simulink model "SSMM_sim_Torque_3DOF"  (R2021a)
settings: Solver=FixedStepAuto  StartTime=0.0  StopTime=15  FixedStep=0.001  MaxStep=1e-1  MinStep=1e-6  RelTol=.05  AbsTol=.05  EnableMultiTasking=on
InitFcn:
  | SSMM_sim_Torque_3DOF_Init
values from neighbouring files (symbols this model uses):
  angVeloSat = 4    [prerun.m]
  CP_Num = CP_Base_Num + CP_Wheels_Num    [JACKAL_dynamic_model.m]
  D = 1000    [JACKAL_dynamic_model.m]
  delay = 0.075    [JACKAL_dynamic_model.m]
  K = 1000000    [JACKAL_dynamic_model.m]
  kd = -0.002    [JACKAL_dynamic_model.m]
  ki = 500    [JACKAL_dynamic_model.m]
  kp = 4    [JACKAL_dynamic_model.m]
  model = floatbase(model)    [JACKAL_dynamic_model.m]
  Mu = .85    (= 0.85)    [JACKAL_dynamic_model.m]
  path = waypoints    [AutoRun.m]
  q_init = [0 0 0 0]'    [JACKAL_dynamic_model.m]
  qd_init = [0 0 0 0]'    [JACKAL_dynamic_model.m]
  realistic_linear_velocity_factor = 0.9782    [JACKAL_dynamic_model.m]
  speed = 2    [prerun.m]
  torque_saturation = 7    [JACKAL_dynamic_model.m]
  wheel_radius = .098    (= 0.098)    [JACKAL_dynamic_model.m]
  wheel_veocity_saturation = 2.2    [JACKAL_dynamic_model.m]
  x_init = [1 0 0 0  0 0 zoff   0 0 0  0 0 0]'    [JACKAL_dynamic_model.m]
undefined symbols (not defined in the file or in its folder): DiscIntNeverNeededParam, Fpt, gcontact, gcPosVel
libraries: simulink x8, fuzblock x3, robotalgslib x1
settings Model: Creator=Sergio  LastModifiedBy=auvsl
settings SolverCC: MaxConsecutiveMinStep=5  AlgebraicLoopSolver=TrustRegion
settings DataIOCC: SaveFormat=Array  SignalLoggingSaveFormat=ModelDataLogs  ReturnWorkspaceOutputs=off
settings OptimizationCC: ExpressionDepthLimit=2147483647  LifeSpan=inf
settings DebuggingCC: UnderspecifiedInitializationDetection=Classic  MergeDetectMultiDrivingBlocksExec=none  SolverPrmCheckMsg=warning  MultiTaskDSMMsg=warning  MultiTaskCondExecSysMsg=none  StateNameClashWarn=warning  SFUnexpectedBacktrackingDiag=warning  SFNoUnconditionalDefaultTransitionDiag=warning  SFExecutionAtInitializationDiag=none  SFMachineParentedDataDiag=warning  ArithmeticOperatorsInVariantConditions=warning
settings HardwareCC: ProdBitPerPointer=32  ProdBitPerSizeT=32  ProdBitPerPtrDiffT=32  ProdLargestAtomicFloat=None  ProdIntDivRoundTo=Undefined  ProdEndianess=Unspecified  ProdWordSize=32  ProdHWDeviceType=32-bit Generic
settings ModelReferenceCC: PropagateSignalLabelsOutOfModel=off
settings SFSimCC: SimUseLocalCustomCode=off  CustomCodeUndefinedFunction=UseInterfaceOnly
settings RTWCC: RTWUseLocalCustomCode=off
settings CodeAppCC: StateflowObjectComments=on
settings GRTTargetCC: TargetLangStandard=C89/C90 (ANSI)
settings ConfigComp: CovMetricSettings=dw  CovSaveCumulativeToWorkspaceVar=on  CovSaveSingleToWorkspaceVar=on  CovExternalEMLEnable=off

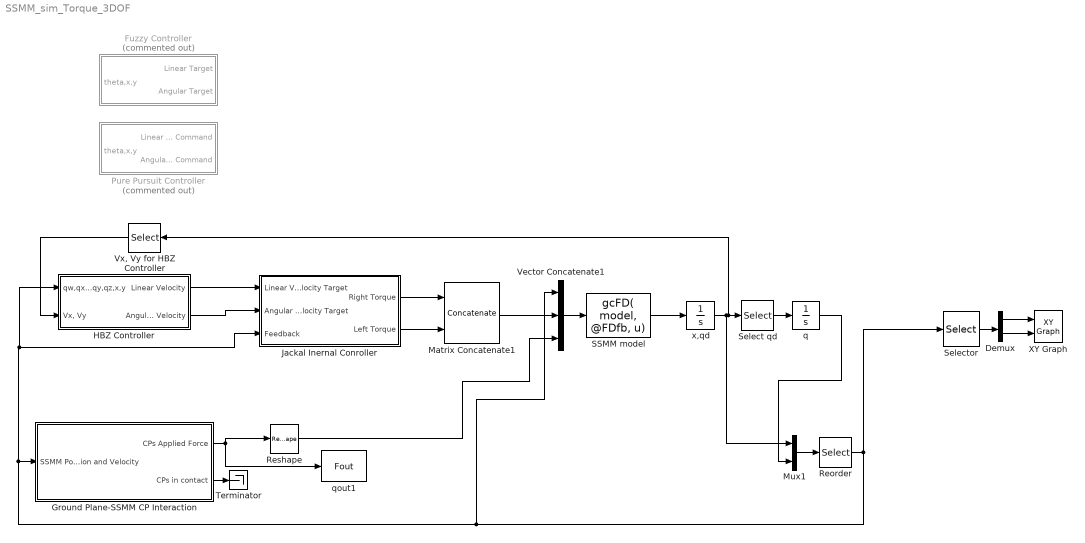
== system SSMM_sim_Torque_3DOF ==
  Demux : Demux  Outputs=2
  Fuzzy Controller : Subsystem  Commented=on
  Ground Plane-SSMM CP Interaction : Subsystem
  HBZ Controller : Subsystem
  Jackal Inernal Conroller : Subsystem
  Matrix Concatenate1 : Concatenate  Mode=Multidimensional array
  Mux1 : Mux  Inputs=2
  Pure Pursuit Controller : Subsystem  Commented=on
  Reorder : Selector  InputPortWidth=21  IndexOptions=Index vector (dialog)  Indices=[1 2 3 4 5 6 7 8 9 10 11 12 13 18 19 20 21 14 15 16 17]  OutputSizes=1
  Reshape : Reshape  OutputDimensionality=Column vector (2-D)
  SSMM model : MATLABFcn  MATLABFcn=gcFD( model, @FDfb, u)  OutputDimensions=[17 1]  OutputSignalType=real  Output1D=off
  Select qd : Selector  InputPortWidth=17  IndexOptions=Index vector (dialog)  Indices=[14 15 16 17]  OutputSizes=1
  Selector : Selector  InputPortWidth=21  IndexOptions=Index vector (dialog)  Indices=[5 6]  OutputSizes=1
  Terminator : Terminator
  Vector Concatenate1 : Concatenate  NumInputs=3
  "Vx, Vy for HBZ Controller" : Selector  InputPortWidth=17  IndexOptions=Index vector (dialog)  Indices=[5, 6]  OutputSizes=1
  XY Graph : simulink/Sinks/XY Graph  xmin=0  xmax=20  ymin=-10  ymax=10  st=-1
  q : Integrator  InitialCondition=q_init
  qout1 : ToWorkspace  VariableName=Fout  SampleTime=-1
  x,qd : Integrator  InitialCondition=[x_init;qd_init]
  wires:
  Vector Concatenate1/1 -> SSMM model/1
  SSMM model/1 -> x,qd/1
  Reshape/1 -> Vector Concatenate1/3
  x,qd/1 -> "Vx, Vy for HBZ Controller"/1, Select qd/1, Mux1/1
  Select qd/1 -> q/1
  Mux1/1 -> Reorder/1
  q/1 -> Mux1/2
  Ground Plane-SSMM CP Interaction/1(CPs Applied Force) -> Reshape/1, qout1/1
  Matrix Concatenate1/1 -> Vector Concatenate1/2
  Jackal Inernal Conroller/1(Right Torque) -> Matrix Concatenate1/1
  Jackal Inernal Conroller/2(Left Torque) -> Matrix Concatenate1/2
  Demux/2 -> XY Graph/2
  Selector/1 -> Demux/1
  Demux/1 -> XY Graph/1
  Ground Plane-SSMM CP Interaction/2(CPs in contact) -> Terminator/1
  Reorder/1 -> Vector Concatenate1/1, HBZ Controller/1(qw,qx,qy,qz,x,y), Jackal Inernal Conroller/3(Feedback), Ground Plane-SSMM CP Interaction/1(SSMM Position and Velocity), Selector/1
  HBZ Controller/1(Linear Velocity) -> Jackal Inernal Conroller/1(Linear Velocity Target)
  HBZ Controller/2(Angular Velocity) -> Jackal Inernal Conroller/2(Angular Velocity Target)
  "Vx, Vy for HBZ Controller"/1 -> HBZ Controller/2("Vx, Vy")

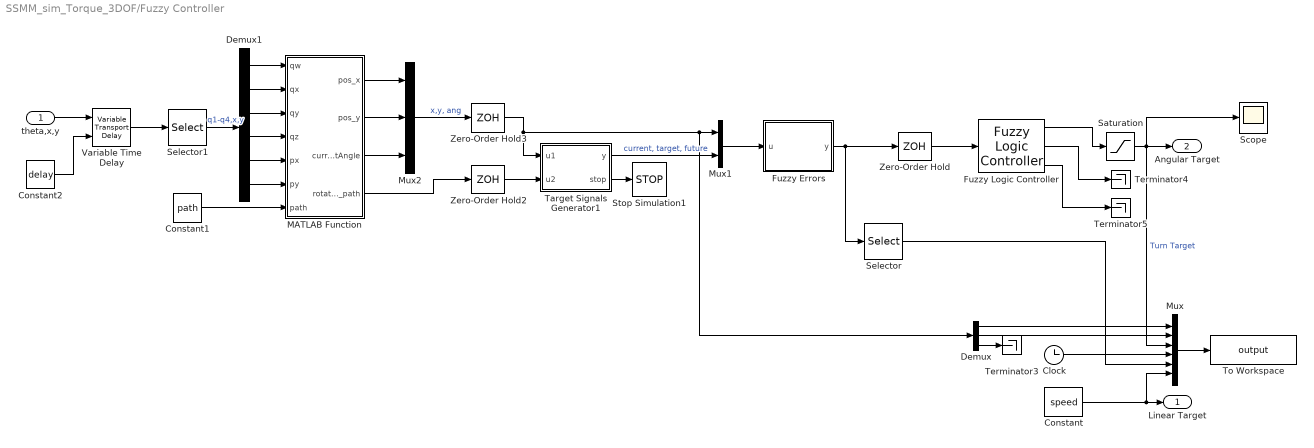
== system SSMM_sim_Torque_3DOF/Fuzzy Controller ==
  theta,x,y : Inport
  Clock : Clock
  Constant : Constant  Value=speed
  Constant1 : Constant  Value=path
  Constant2 : Constant  Value=delay
  Demux : Demux  Outputs=3
  Demux1 : Demux  Outputs=6
  Fuzzy Errors : MATLAB Function  TreatAsAtomicUnit=on
  Fuzzy Logic Controller : fuzblock/Fuzzy Logic  Controller  FIS='fuzV1.fis'  OutputSampleNumber=3000  DataType=double  FuzzifiedInputs=off  RuleFiringStrengths=on  RuleOutputs=off  AggregatedOutputs=on  SimulateUsing=Code generation  OutOfRangeInputValueMessage=warning  NoRuleFiredMessage=warning  EmptyOutputFuzzySetMessage=warning
  MATLAB Function : MATLAB Function  TreatAsAtomicUnit=on
  Mux : Mux  Inputs=6
  Mux1 : Mux  Inputs=2
  Mux2 : Mux  Inputs=3
  Saturation : Saturate  UpperLimit=angVeloSat  LowerLimit=-angVeloSat
  Scope : Scope
  Selector : Selector  InputPortWidth=5  IndexOptions=Index vector (dialog)  Indices=[1]  OutputSizes=1
  Selector1 : Selector  InputPortWidth=21  IndexOptions=Index vector (dialog)  Indices=[1 2 3 4 5 6]  OutputSizes=1
  Stop Simulation1 : Stop
  Target Signals Generator1 : MATLAB Function  TreatAsAtomicUnit=on
  Terminator3 : Terminator
  Terminator4 : Terminator
  Terminator5 : Terminator
  To Workspace : ToWorkspace  VariableName=output  SampleTime=-1
  Variable Time Delay : VariableTransportDelay  MaximumDelay=10  MaximumPoints=6244
  Zero-Order Hold : ZeroOrderHold  SampleTime=.001
  Zero-Order Hold2 : ZeroOrderHold  SampleTime=.001
  Zero-Order Hold3 : ZeroOrderHold  SampleTime=.001
  Linear Target : Outport  VectorParamsAs1DForOutWhenUnconnected=off
  " Angular Target" : Outport  Port=2  VectorParamsAs1DForOutWhenUnconnected=off
  wires:
  Mux1/1 -> Fuzzy Errors/1(u)
  Target Signals Generator1/1(y) -> Mux1/2  "current, target, future"
  Zero-Order Hold2/1 -> Target Signals Generator1/2(u2)
  Target Signals Generator1/2(stop) -> Stop Simulation1/1
  Fuzzy Errors/1(y) -> Selector/1, Zero-Order Hold/1
  Zero-Order Hold/1 -> Fuzzy Logic Controller/1
  Fuzzy Logic Controller/1 -> Saturation/1
  Saturation/1 -> Scope/1, Mux/3, " Angular Target"/1  "Turn Target"
  theta,x,y/1 -> Variable Time Delay/1
  Variable Time Delay/1 -> Selector1/1
  Constant/1 -> Mux/6, Linear Target/1
  Selector/1 -> Mux/5
  Mux/1 -> To Workspace/1
  Zero-Order Hold3/1 -> Target Signals Generator1/1(u1), Mux1/1, Demux/1
  Constant2/1 -> Variable Time Delay/2
  Clock/1 -> Mux/4
  Fuzzy Logic Controller/2 -> Terminator4/1
  Fuzzy Logic Controller/3 -> Terminator5/1
  MATLAB Function/3(currentAngle) -> Mux2/3
  MATLAB Function/1(pos_x) -> Mux2/1
  MATLAB Function/2(pos_y) -> Mux2/2
  MATLAB Function/4(rotated_path) -> Zero-Order Hold2/1
  Mux2/1 -> Zero-Order Hold3/1  "x,y, ang"
  Constant1/1 -> MATLAB Function/7(path)
  Demux1/1 -> MATLAB Function/1(qw)
  Demux1/2 -> MATLAB Function/2(qx)
  Demux1/3 -> MATLAB Function/3(qy)
  Demux1/4 -> MATLAB Function/4(qz)
  Demux1/5 -> MATLAB Function/5(px)
  Demux1/6 -> MATLAB Function/6(py)
  Selector1/1 -> Demux1/1  "q1-q4,x,y"
  Demux/3 -> Terminator3/1
  Demux/2 -> Mux/2
  Demux/1 -> Mux/1

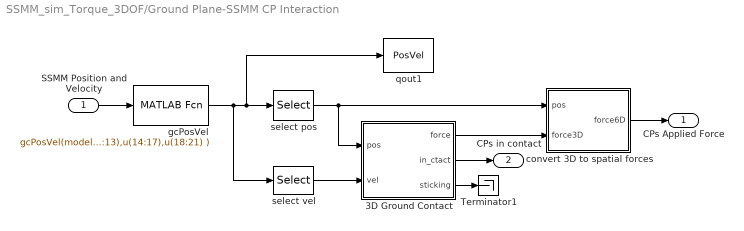
== system SSMM_sim_Torque_3DOF/Ground Plane-SSMM CP Interaction ==
  SSMM Position and Velocity : Inport
  3D Ground Contact : Subsystem  mask(3D Nonlinear Ground Contact with Friction){K=K, D=D, mu=Mu, np=CP_Num}
      mask prompts: K "Stiffness (K)"; D "Damping (D)"; mu "Coefficient of Friction (mu)"; np "Number of Contact Points"
      mask help:
      | Given two 3xnp arrays containing contact-point positions and
      | velocities, calculate the 3xnp array of ground-reaction forces
      | acting on those points. Also calculate 1xnp boolean vectors
      | in_ctact (true if normal force >0) and sticking (true if inside
      | or on boundary of friction cone).  Zero-crossing detection is
      | enabled at both make/break contact and stick/slip transitions.
  Terminator1 : Terminator
  convert 3D to spatial forces : Subsystem
  gcPosVel : MATLABFcn  MATLABFcn=gcPosVel(model, u(1:13),u(14:17),u(18:21) )  OutputDimensions=[6 CP_Num]  OutputSignalType=real  Output1D=off
  qout1 : ToWorkspace  VariableName=PosVel  SampleTime=-1
  select pos : Selector  NumberOfDimensions=2  InputPortWidth=3  IndexOptions=Index vector (dialog),Select all  Indices=[1 2 3],1  OutputSizes=1,1
  select vel : Selector  NumberOfDimensions=2  InputPortWidth=3  IndexOptions=Index vector (dialog),Select all  Indices=[4 5 6],1  OutputSizes=1,1
  CPs Applied Force : Outport  VectorParamsAs1DForOutWhenUnconnected=off
  CPs in contact : Outport  Port=2  VectorParamsAs1DForOutWhenUnconnected=off
  wires:
  gcPosVel/1 -> select vel/1, qout1/1, select pos/1
  select pos/1 -> convert 3D to spatial forces/1(pos), 3D Ground Contact/1(pos)
  convert 3D to spatial forces/1(force6D) -> CPs Applied Force/1
  select vel/1 -> 3D Ground Contact/2(vel)
  3D Ground Contact/3(sticking) -> Terminator1/1
  3D Ground Contact/2(in_ctact) -> CPs in contact/1
  SSMM Position and Velocity/1 -> gcPosVel/1
  3D Ground Contact/1(force) -> convert 3D to spatial forces/2(force3D)

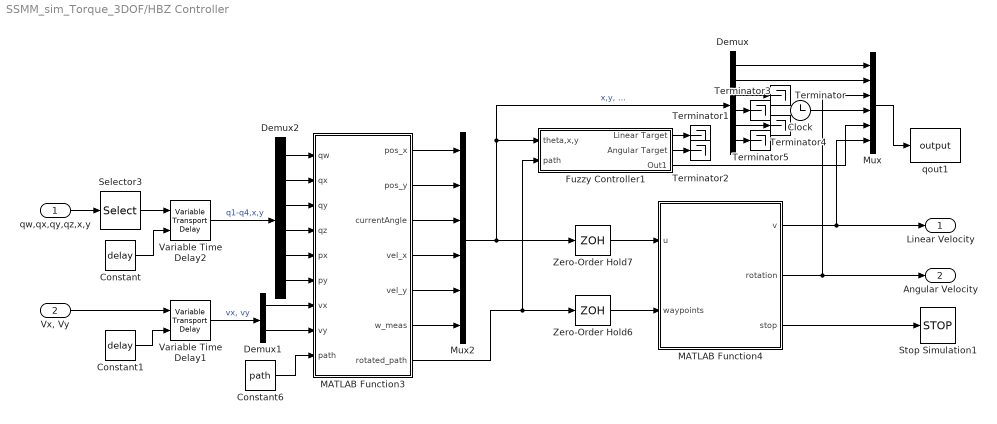
== system SSMM_sim_Torque_3DOF/HBZ Controller ==
  qw,qx,qy,qz,x,y : Inport
  "Vx, Vy" : Inport  Port=2
  Clock : Clock
  Constant : Constant  Value=delay
  Constant1 : Constant  Value=delay
  Constant6 : Constant  Value=path
  Demux : Demux  Outputs=6
  Demux1 : Demux  Outputs=2
  Demux2 : Demux  Outputs=6
  Fuzzy Controller1 : Subsystem
  MATLAB Function3 : MATLAB Function  TreatAsAtomicUnit=on
  MATLAB Function4 : MATLAB Function  TreatAsAtomicUnit=on
  Mux : Mux  Inputs=6
  Mux2 : Mux  Inputs=6
  Selector3 : Selector  InputPortWidth=21  IndexOptions=Index vector (dialog)  Indices=[1 2 3 4 5 6]  OutputSizes=1
  Stop Simulation1 : Stop
  Terminator{,1..5} (6 alike) : Terminator
  Variable Time Delay1 : VariableTransportDelay  MaximumDelay=10  MaximumPoints=10340
  Variable Time Delay2 : VariableTransportDelay  MaximumDelay=10  MaximumPoints=10340
  Zero-Order Hold6 : ZeroOrderHold  SampleTime=-1
  Zero-Order Hold7 : ZeroOrderHold  SampleTime=-1
  qout1 : ToWorkspace  VariableName=output  SampleTime=-1
  Linear Velocity : Outport  VectorParamsAs1DForOutWhenUnconnected=off
  Angular Velocity : Outport  Port=2  VectorParamsAs1DForOutWhenUnconnected=off
  wires:
  Demux/1 -> Mux/1
  MATLAB Function4/1(v) -> Linear Velocity/1, Mux/6
  MATLAB Function3/2(pos_y) -> Mux2/2
  MATLAB Function3/1(pos_x) -> Mux2/1
  Demux/3 -> Terminator/1
  Zero-Order Hold7/1 -> MATLAB Function4/1(u)
  Demux/2 -> Mux/2
  Mux2/1 -> Fuzzy Controller1/1(theta,x,y), Demux/1, Zero-Order Hold7/1  "x,y, ..."
  Fuzzy Controller1/1(Linear Target) -> Terminator1/1
  qw,qx,qy,qz,x,y/1 -> Selector3/1
  Demux2/3 -> MATLAB Function3/3(qy)
  Mux/1 -> qout1/1
  Demux2/5 -> MATLAB Function3/5(px)
  Demux2/2 -> MATLAB Function3/2(qx)
  Constant6/1 -> MATLAB Function3/9(path)
  MATLAB Function3/7(rotated_path) -> Fuzzy Controller1/2(path), Zero-Order Hold6/1
  Constant/1 -> Variable Time Delay2/2
  Demux2/6 -> MATLAB Function3/6(py)
  Variable Time Delay2/1 -> Demux2/1  "q1-q4,x,y"
  Demux2/4 -> MATLAB Function3/4(qz)
  MATLAB Function3/3(currentAngle) -> Mux2/3
  Selector3/1 -> Variable Time Delay2/1
  Demux2/1 -> MATLAB Function3/1(qw)
  Clock/1 -> Mux/4
  Fuzzy Controller1/3(Out1) -> Mux/5
  MATLAB Function4/2(rotation) -> Angular Velocity/1, Mux/3
  Zero-Order Hold6/1 -> MATLAB Function4/2(waypoints)
  Fuzzy Controller1/2(" Angular Target") -> Terminator2/1
  Constant1/1 -> Variable Time Delay1/2
  "Vx, Vy"/1 -> Variable Time Delay1/1
  Variable Time Delay1/1 -> Demux1/1  "vx, vy"
  Demux1/2 -> MATLAB Function3/8(vy)
  Demux1/1 -> MATLAB Function3/7(vx)
  MATLAB Function3/4(vel_x) -> Mux2/4
  MATLAB Function3/5(vel_y) -> Mux2/5
  MATLAB Function3/6(w_meas) -> Mux2/6
  MATLAB Function4/3(stop) -> Stop Simulation1/1
  Demux/4 -> Terminator3/1
  Demux/5 -> Terminator4/1
  Demux/6 -> Terminator5/1

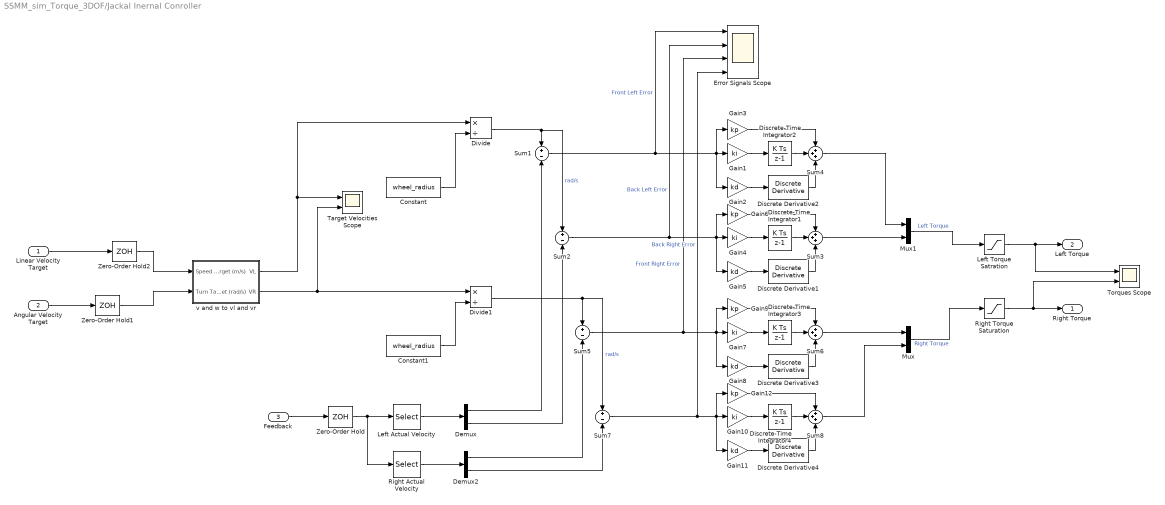
== system SSMM_sim_Torque_3DOF/Jackal Inernal Conroller ==
  Linear Velocity Target : Inport
  Angular Velocity Target : Inport  Port=2
  Feedback : Inport  Port=3
  Constant : Constant  Value=wheel_radius
  Constant1 : Constant  Value=wheel_radius
  Demux : Demux  Outputs=2
  Demux2 : Demux  Outputs=2
  Discrete Derivative{1..4} (4 alike) : simulink/Discrete/Discrete Derivative  gainval=1  ICPrevScaledInput=0.0  OutMin=[]  OutMax=[]  OutDataType=fixdt(1, 16)  OutScaling=2^-10  DoSatur=off
  Discrete-Time Integrator{1..4} (4 alike) : DiscreteIntegrator  SampleTime=-1  ICPrevOutput=DiscIntNeverNeededParam  ICPrevScaledInput=DiscIntNeverNeededParam
  Divide : Product  Inputs=*/
  Divide1 : Product  Inputs=*/
  Error Signals Scope : Scope  NumInputPorts=4
  Gain{1,4,7,10} (4 alike) : Gain  Gain=ki
  Gain{2,5,8,11} (4 alike) : Gain  Gain=kd
  Gain{3,6,9,12} (4 alike) : Gain  Gain=kp
  Left Actual Velocity : Selector  InputPortWidth=21  IndexOptions=Index vector (dialog)  Indices=[20 21]  OutputSizes=1
  Left Torque Satration : Saturate  UpperLimit=torque_saturation  LowerLimit=-torque_saturation
  Mux : Mux  Inputs=2
  Mux1 : Mux  Inputs=2
  Right Actual Velocity : Selector  InputPortWidth=21  IndexOptions=Index vector (dialog)  Indices=[18 19]  OutputSizes=1
  Right Torque Saturation : Saturate  UpperLimit=torque_saturation  LowerLimit=-torque_saturation
  Sum{1..2,5,7} (4 alike) : Sum  Inputs=+-
  Sum{3..4,6,8} (4 alike) : Sum  Inputs=+++
  Target Velocities Scope : Scope  NumInputPorts=2
  Torques Scope : Scope  NumInputPorts=2
  Zero-Order Hold : ZeroOrderHold  SampleTime=-1
  Zero-Order Hold1 : ZeroOrderHold  SampleTime=-1
  Zero-Order Hold2 : ZeroOrderHold  SampleTime=-1
  v and w to vl and vr : Subsystem
  Right Torque : Outport  VectorParamsAs1DForOutWhenUnconnected=off
  Left Torque : Outport  Port=2  VectorParamsAs1DForOutWhenUnconnected=off
  wires:
  Feedback/1 -> Zero-Order Hold/1
  Constant/1 -> Divide/2
  Constant1/1 -> Divide1/2
  Zero-Order Hold/1 -> Right Actual Velocity/1, Left Actual Velocity/1
  v and w to vl and vr/1(VL) -> Target Velocities Scope/1, Divide/1
  Right Torque Saturation/1 -> Torques Scope/2, Right Torque/1
  Discrete Derivative2/1 -> Sum4/3
  Sum1/1 -> Error Signals Scope/1, Gain3/1, Gain2/1, Gain1/1  "Front Left Error"
  Sum4/1 -> Mux1/1
  Discrete-Time Integrator2/1 -> Sum4/2
  Gain3/1 -> Sum4/1
  Gain2/1 -> Discrete Derivative2/1
  Gain1/1 -> Discrete-Time Integrator2/1
  Discrete-Time Integrator1/1 -> Sum3/2
  Gain4/1 -> Discrete-Time Integrator1/1
  Gain5/1 -> Discrete Derivative1/1
  Sum3/1 -> Mux1/2
  Sum2/1 -> Error Signals Scope/2, Gain6/1, Gain5/1, Gain4/1  "Back Left Error"
  Gain6/1 -> Sum3/1
  Discrete Derivative1/1 -> Sum3/3
  Discrete-Time Integrator3/1 -> Sum6/2
  Gain7/1 -> Discrete-Time Integrator3/1
  Gain8/1 -> Discrete Derivative3/1
  Sum5/1 -> Error Signals Scope/3, Gain9/1, Gain8/1, Gain7/1  "Front Right Error"
  Gain9/1 -> Sum6/1
  Discrete Derivative3/1 -> Sum6/3
  Discrete-Time Integrator4/1 -> Sum8/2
  Gain10/1 -> Discrete-Time Integrator4/1
  Gain11/1 -> Discrete Derivative4/1
  Sum7/1 -> Error Signals Scope/4, Gain10/1, Gain12/1, Gain11/1  "Back Right Error"
  Gain12/1 -> Sum8/1
  Discrete Derivative4/1 -> Sum8/3
  Mux1/1 -> Left Torque Satration/1  "Left Torque"
  Left Torque Satration/1 -> Torques Scope/1, Left Torque/1
  Mux/1 -> Right Torque Saturation/1  "Right Torque"
  Sum6/1 -> Mux/1
  Sum8/1 -> Mux/2
  Right Actual Velocity/1 -> Demux2/1
  Left Actual Velocity/1 -> Demux/1
  Demux2/2 -> Sum7/2
  Demux2/1 -> Sum5/2
  Demux/2 -> Sum2/2
  Demux/1 -> Sum1/2
  Angular Velocity Target/1 -> Zero-Order Hold1/1
  v and w to vl and vr/2(VR) -> Target Velocities Scope/2, Divide1/1
  Divide1/1 -> Sum7/1, Sum5/1  "rad/s"
  Divide/1 -> Sum2/1, Sum1/1  "rad/s"
  Zero-Order Hold2/1 -> v and w to vl and vr/1(Speed Target (m/s))
  Zero-Order Hold1/1 -> v and w to vl and vr/2(Turn Target (rad/s))
  Linear Velocity Target/1 -> Zero-Order Hold2/1

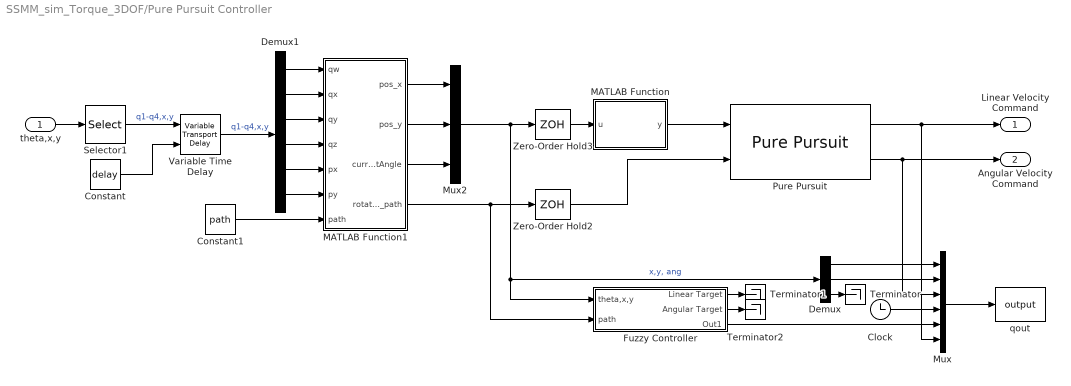
== system SSMM_sim_Torque_3DOF/Pure Pursuit Controller ==
  theta,x,y : Inport
  Clock : Clock
  Constant : Constant  Value=delay
  Constant1 : Constant  Value=path
  Demux : Demux  Outputs=3
  Demux1 : Demux  Outputs=6
  Fuzzy Controller : Subsystem
  MATLAB Function : MATLAB Function  TreatAsAtomicUnit=on
  MATLAB Function1 : MATLAB Function  TreatAsAtomicUnit=on
  Mux : Mux  Inputs=6
  Mux2 : Mux  Inputs=3
  Pure Pursuit : robotalgslib/Pure Pursuit  DesiredLinearVelocity=speed  MaxAngularVelocity=angVeloSat  LookaheadDistance=lookahead  TargetDirPort=off  SimulateUsing=Code generation
  Selector1 : Selector  InputPortWidth=21  IndexOptions=Index vector (dialog)  Indices=[1 2 3 4 5 6]  OutputSizes=1
  Terminator : Terminator
  Terminator1 : Terminator
  Terminator2 : Terminator
  Variable Time Delay : VariableTransportDelay  MaximumDelay=10  MaximumPoints=6244
  Zero-Order Hold2 : ZeroOrderHold  SampleTime=.001
  Zero-Order Hold3 : ZeroOrderHold  SampleTime=.001
  qout : ToWorkspace  VariableName=output  SampleTime=-1
  Linear Velocity Command : Outport  VectorParamsAs1DForOutWhenUnconnected=off
  Angular Velocity Command : Outport  Port=2  VectorParamsAs1DForOutWhenUnconnected=off
  wires:
  Zero-Order Hold3/1 -> MATLAB Function/1(u)
  Selector1/1 -> Variable Time Delay/1  "q1-q4,x,y"
  theta,x,y/1 -> Selector1/1
  MATLAB Function/1(y) -> Pure Pursuit/1
  Zero-Order Hold2/1 -> Pure Pursuit/2
  Pure Pursuit/2 -> Mux/3, Angular Velocity Command/1
  Pure Pursuit/1 -> Mux/6, Linear Velocity Command/1
  Constant/1 -> Variable Time Delay/2
  Mux/1 -> qout/1
  Clock/1 -> Mux/4
  Fuzzy Controller/3(Out1) -> Mux/5
  Demux/1 -> Mux/1
  Demux/2 -> Mux/2
  Demux/3 -> Terminator/1
  Fuzzy Controller/1(Linear Target) -> Terminator1/1
  Fuzzy Controller/2(" Angular Target") -> Terminator2/1
  Demux1/2 -> MATLAB Function1/2(qx)
  Variable Time Delay/1 -> Demux1/1  "q1-q4,x,y"
  MATLAB Function1/4(rotated_path) -> Fuzzy Controller/2(path), Zero-Order Hold2/1
  Demux1/3 -> MATLAB Function1/3(qy)
  Demux1/5 -> MATLAB Function1/5(px)
  MATLAB Function1/3(currentAngle) -> Mux2/3
  Mux2/1 -> Demux/1, Fuzzy Controller/1(theta,x,y), Zero-Order Hold3/1  "x,y, ang"
  MATLAB Function1/2(pos_y) -> Mux2/2
  Demux1/4 -> MATLAB Function1/4(qz)
  MATLAB Function1/1(pos_x) -> Mux2/1
  Demux1/6 -> MATLAB Function1/6(py)
  Demux1/1 -> MATLAB Function1/1(qw)
  Constant1/1 -> MATLAB Function1/7(path)

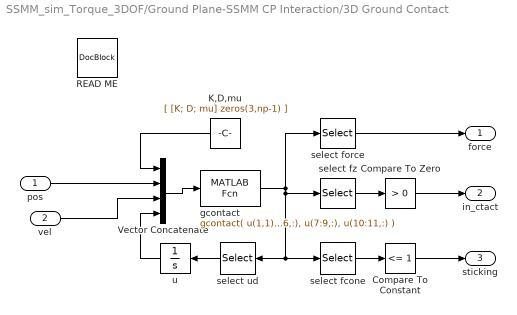
== system SSMM_sim_Torque_3DOF/Ground Plane-SSMM CP Interaction/3D Ground Contact ==
  pos : Inport
  vel : Inport  Port=2
  Compare To Constant : simulink/Logic and Bit Operations/Compare To Constant  relop=<=  const=1  OutDataTypeStr=boolean
  Compare To Zero : simulink/Logic and Bit Operations/Compare To Zero  relop=>  OutDataTypeStr=boolean
  K,D,mu : Constant  Value=[ [K; D; mu] zeros(3,np-1) ]  VectorParams1D=off
  READ ME : simulink/Model-Wide Utilities/DocBlock  DocumentType=Text
      content=|
      | The constant block supplies the parameters K, D and mu to the function
      | gcontact.  This is necessary because K, D and mu are defined in the
      | workspace of this particular masked subsystem, but the executable
      | expression in the "MATLAB Function" block does not have access to this
      | workspace, so the symbols K, D and mu cannot appear directly in the
      | executable expression.
      |
      | The ">0" block and the "<=1" block both have zero-crossing enabled.  The
      | former detects transitions between contact and non-contact, whereas the
      | latter detects transitions between sticking (due to friction) and
      | slipping.  A point can be sticking only if it is also in contact.  A
      | zero-crossing event occurs whenever any one point makes a transition.
      |
      | The state variable, u, is a 2x(np) matrix containing the horizontal
      | component of the local ground deformation for each point.  This quantity
      | is used to calculate the tangential (i.e., frictional) component of the
      | ground reaction force.
      |
      | When a point loses contact, its associated state variable, u(:,i), decays
      | to zero with a time constant of D/K.  If this ratio is small then the
      | corresponding differential equation is fast, and it is necessary to use
      | small integration time steps.  For example, if K=1e6 and D=2000 then
      | D/K=0.002 and u(:,i) decays in proportion to exp(-500t).  Increasing K
      | makes the surface stiffer, and decreasing D/K makes it bouncier, but the
      | latter also makes the post-contact recovery faster.  The degree of
      | bounciness depends on the mass of the impacting body: a heavier body will
      | bounce more.
      |
      | To adapt this subsystem to work in 2D, the only things that change are the
      | row dimensions of various matrices.  You will have to alter the row
      | selections in the executable expression in the "MATLAB Function" block,
      | and also the dimensions of its output matrix, and you will have to change
      | the row selections in the various "select" blocks.
      |
      | For more information, see "The Simulink Ground Contact Model" in the
      | spatial_v2 documentation directory.
  Vector Concatenate : Concatenate  NumInputs=4  Mode=Multidimensional array
  gcontact : MATLABFcn  MATLABFcn=gcontact( u(1,1), u(2,1), u(3,1), u(4:6,:), u(7:9,:), u(10:11,:) )  OutputDimensions=[6 np]  OutputSignalType=real  Output1D=off
  select fcone : Selector  NumberOfDimensions=2  InputPortWidth=3  IndexOptions=Index vector (dialog),Select all  Indices=[6],1  OutputSizes=1,1
  select force : Selector  NumberOfDimensions=2  InputPortWidth=3  IndexOptions=Index vector (dialog),Select all  Indices=[1 2 3],1  OutputSizes=1,1
  select fz : Selector  NumberOfDimensions=2  InputPortWidth=3  IndexOptions=Index vector (dialog),Select all  Indices=[3],1  OutputSizes=1,1
  select ud : Selector  NumberOfDimensions=2  InputPortWidth=3  IndexOptions=Index vector (dialog),Select all  Indices=[4 5],1  OutputSizes=1,1
  u : Integrator
  force : Outport  VectorParamsAs1DForOutWhenUnconnected=off
  in_ctact : Outport  Port=2  VectorParamsAs1DForOutWhenUnconnected=off
  sticking : Outport  Port=3  VectorParamsAs1DForOutWhenUnconnected=off
  wires:
  Vector Concatenate/1 -> gcontact/1
  select ud/1 -> u/1
  gcontact/1 -> select fz/1, select ud/1, select fcone/1, select force/1
  select fz/1 -> Compare To Zero/1
  select fcone/1 -> Compare To Constant/1
  Compare To Constant/1 -> sticking/1
  u/1 -> Vector Concatenate/4
  pos/1 -> Vector Concatenate/2
  K,D,mu/1 -> Vector Concatenate/1
  vel/1 -> Vector Concatenate/3
  Compare To Zero/1 -> in_ctact/1
  select force/1 -> force/1

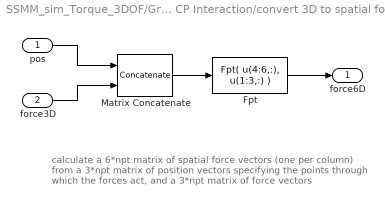
== system SSMM_sim_Torque_3DOF/Ground Plane-SSMM CP Interaction/convert 3D to spatial forces ==
  note: calculate a 6*npt matrix of spatial force vectors (one per column)
      | from a 3*npt matrix of position vectors specifying the points
      | through which the forces act, and a 3*npt matrix of force vectors
  pos : Inport
  force3D : Inport  Port=2
  Fpt : MATLABFcn  MATLABFcn=Fpt( u(4:6,:), u(1:3,:) )  OutputSignalType=real  Output1D=off
  Matrix Concatenate : Concatenate  Mode=Multidimensional array
  force6D : Outport  VectorParamsAs1DForOutWhenUnconnected=off
  wires:
  force3D/1 -> Matrix Concatenate/2
  pos/1 -> Matrix Concatenate/1
  Matrix Concatenate/1 -> Fpt/1
  Fpt/1 -> force6D/1

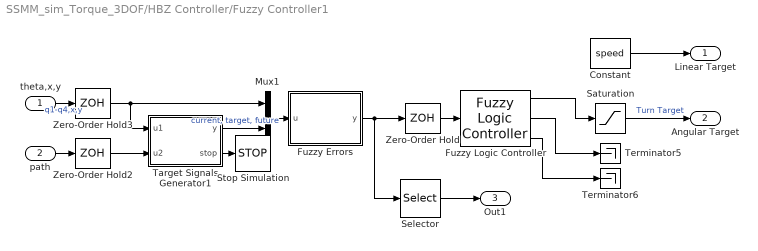
== system SSMM_sim_Torque_3DOF/HBZ Controller/Fuzzy Controller1 ==
  theta,x,y : Inport
  path : Inport  Port=2
  Constant : Constant  Value=speed
  Fuzzy Errors : MATLAB Function  TreatAsAtomicUnit=on
  Fuzzy Logic Controller : fuzblock/Fuzzy Logic  Controller  FIS='fuzzyControl.fis'  OutputSampleNumber=3000  DataType=double  FuzzifiedInputs=off  RuleFiringStrengths=on  RuleOutputs=off  AggregatedOutputs=on  SimulateUsing=Code generation  OutOfRangeInputValueMessage=warning  NoRuleFiredMessage=warning  EmptyOutputFuzzySetMessage=warning
  Mux1 : Mux  Inputs=2
  Saturation : Saturate  UpperLimit=angVeloSat  LowerLimit=-angVeloSat
  Selector : Selector  InputPortWidth=5  IndexOptions=Index vector (dialog)  Indices=[1]  OutputSizes=1
  Stop Simulation : Stop
  Target Signals Generator1 : MATLAB Function  TreatAsAtomicUnit=on
  Terminator5 : Terminator
  Terminator6 : Terminator
  Zero-Order Hold : ZeroOrderHold  SampleTime=-1
  Zero-Order Hold2 : ZeroOrderHold  SampleTime=-1
  Zero-Order Hold3 : ZeroOrderHold  SampleTime=-1
  Linear Target : Outport  VectorParamsAs1DForOutWhenUnconnected=off
  " Angular Target" : Outport  Port=2  VectorParamsAs1DForOutWhenUnconnected=off
  Out1 : Outport  Port=3
  wires:
  Mux1/1 -> Fuzzy Errors/1(u)
  Target Signals Generator1/1(y) -> Mux1/2  "current, target, future"
  path/1 -> Zero-Order Hold2/1
  Zero-Order Hold2/1 -> Target Signals Generator1/2(u2)
  Fuzzy Errors/1(y) -> Selector/1, Zero-Order Hold/1
  Zero-Order Hold/1 -> Fuzzy Logic Controller/1
  Fuzzy Logic Controller/1 -> Saturation/1
  Constant/1 -> Linear Target/1
  theta,x,y/1 -> Zero-Order Hold3/1  "q1-q4,x,y"
  Zero-Order Hold3/1 -> Target Signals Generator1/1(u1), Mux1/1
  Saturation/1 -> " Angular Target"/1  "Turn Target"
  Selector/1 -> Out1/1
  Fuzzy Logic Controller/2 -> Terminator5/1
  Fuzzy Logic Controller/3 -> Terminator6/1
  Target Signals Generator1/2(stop) -> Stop Simulation/1

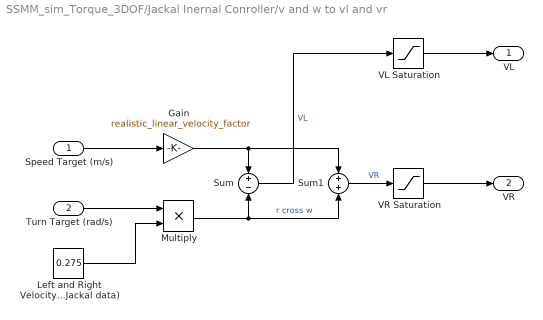
== system SSMM_sim_Torque_3DOF/Jackal Inernal Conroller/v and w to vl and vr ==
  Speed Target (m/s) : Inport
      settings: AttributesFormatString=Speed Target (m/s)
  Turn Target (rad/s) : Inport  Port=2
  Gain : Gain  Gain=realistic_linear_velocity_factor
  Left and Right Velocity Assignment constant (determined from real-Jackal data) : Constant  Value=0.275
  Multiply : Product  Inputs=**
  Sum : Sum  Inputs=+|-
  Sum1 : Sum  Inputs=+|+
  VL Saturation : Saturate  UpperLimit=wheel_veocity_saturation  LowerLimit=-wheel_veocity_saturation
  VR Saturation : Saturate  UpperLimit=wheel_veocity_saturation  LowerLimit=-wheel_veocity_saturation
  VL : Outport  VectorParamsAs1DForOutWhenUnconnected=off
  VR : Outport  Port=2  VectorParamsAs1DForOutWhenUnconnected=off
  wires:
  Multiply/1 -> Sum/2, Sum1/2  "r cross w"
  Speed Target (m/s)/1 -> Gain/1
  Sum/1 -> VL Saturation/1  "VL"
  Sum1/1 -> VR Saturation/1  "VR"
  VR Saturation/1 -> VR/1
  Turn Target (rad/s)/1 -> Multiply/1
  Left and Right Velocity Assignment constant (determined from real-Jackal data)/1 -> Multiply/2
  VL Saturation/1 -> VL/1
  Gain/1 -> Sum1/1, Sum/1

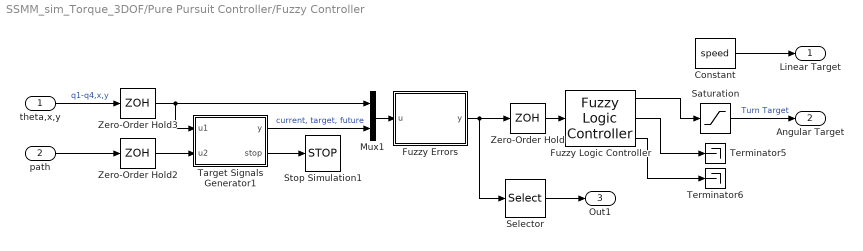
== system SSMM_sim_Torque_3DOF/Pure Pursuit Controller/Fuzzy Controller ==
  theta,x,y : Inport
  path : Inport  Port=2
  Constant : Constant  Value=speed
  Fuzzy Errors : MATLAB Function  TreatAsAtomicUnit=on
  Fuzzy Logic Controller : fuzblock/Fuzzy Logic  Controller  FIS='fuzzyControl.fis'  OutputSampleNumber=3000  DataType=double  FuzzifiedInputs=off  RuleFiringStrengths=on  RuleOutputs=off  AggregatedOutputs=on  SimulateUsing=Code generation  OutOfRangeInputValueMessage=warning  NoRuleFiredMessage=warning  EmptyOutputFuzzySetMessage=warning
  Mux1 : Mux  Inputs=2
  Saturation : Saturate  UpperLimit=angVeloSat  LowerLimit=-angVeloSat
  Selector : Selector  InputPortWidth=5  IndexOptions=Index vector (dialog)  Indices=[1]  OutputSizes=1
  Stop Simulation1 : Stop
  Target Signals Generator1 : MATLAB Function  TreatAsAtomicUnit=on
  Terminator5 : Terminator
  Terminator6 : Terminator
  Zero-Order Hold : ZeroOrderHold  SampleTime=.001
  Zero-Order Hold2 : ZeroOrderHold  SampleTime=.001
  Zero-Order Hold3 : ZeroOrderHold  SampleTime=.001
  Linear Target : Outport  VectorParamsAs1DForOutWhenUnconnected=off
  " Angular Target" : Outport  Port=2  VectorParamsAs1DForOutWhenUnconnected=off
  Out1 : Outport  Port=3
  wires:
  Mux1/1 -> Fuzzy Errors/1(u)
  Target Signals Generator1/1(y) -> Mux1/2  "current, target, future"
  path/1 -> Zero-Order Hold2/1
  Zero-Order Hold2/1 -> Target Signals Generator1/2(u2)
  Target Signals Generator1/2(stop) -> Stop Simulation1/1
  Fuzzy Errors/1(y) -> Selector/1, Zero-Order Hold/1
  Zero-Order Hold/1 -> Fuzzy Logic Controller/1
  Fuzzy Logic Controller/1 -> Saturation/1
  Constant/1 -> Linear Target/1
  theta,x,y/1 -> Zero-Order Hold3/1  "q1-q4,x,y"
  Zero-Order Hold3/1 -> Target Signals Generator1/1(u1), Mux1/1
  Saturation/1 -> " Angular Target"/1  "Turn Target"
  Selector/1 -> Out1/1
  Fuzzy Logic Controller/2 -> Terminator5/1
  Fuzzy Logic Controller/3 -> Terminator6/1

== matlab function SSMM_sim_Torque_3DOF/HBZ Controller/Fuzzy Controller1/Target Signals Generator1 ==
  data: u1 input; y output; u2 input; stop output
function [y,stop] = fcn(u1,u2)
persistent pathcount;
persistent pathlength;
persistent path; %error in code, initially used path but this is already a matlab function
persistent pathPre;

if isempty(pathcount)
   pathcount=1;
   pathPre=u2;
   [pathlength,~]=size(pathPre);  
   path=[pathPre; pathPre(pathlength,1)+100 pathPre(pathlength,2)+100]; %sim takes multiple iterations to stop after reaching final point, so this prevents it from breaking
end


pos=[u1(1) u1(2)]; % [x,y] 
currentPoint=path(pathcount,:);
target=path(pathcount+1,:);

A = [(currentPoint(2)-target(2)), target(1)-currentPoint(1); target(1)-currentPoint(1), target(2)-currentPoint(2)];
b = [ target(1)*currentPoint(2)-currentPoint(1)*target(2); pos(1)*(target(1)-currentPoint(1)) + pos(2)*(target(2)-currentPoint(2))];
proj = (A\b)'; %projected point on the line between  .
projLen=dot(proj-currentPoint,target-currentPoint)/norm(target-currentPoint)^2; %the distance along the projected line, where 0 is the start point and 1 is the end point

if ((projLen>1))
    pathcount=pathcount+1;
end

pathflag=0;
if (pathcount==pathlength)
    pathflag=1;
end
stop = pathflag;
if ((pathcount==(pathlength-1))||(pathcount==(pathlength)))
    a=path(pathcount,:);
    b=path(pathcount+1,:);
    diff = (b-a) / norm(b-a);
    post = b + diff;
else
    a=path(pathcount,:);
    b=path(pathcount+1,:);
    post=path(pathcount+2,:);
end

y = [a(1);a(2);b(1);b(2);post(1);post(2)];

== matlab function SSMM_sim_Torque_3DOF/HBZ Controller/MATLAB Function3 ==
  data: pos_x output; pos_y output; qw input; currentAngle output; vel_x output; vel_y output; w_meas output; qx input; qy input; qz input; px input; py input; vx input; vy input; path input; rotated_path output
function [pos_x, pos_y, currentAngle, vel_x, vel_y, w_meas, rotated_path] = fcn(qw, qx, qy, qz, px, py, vx, vy, path)
    pos_x = px;
    pos_y = py;
    currentAngle = atan2(2*(qw*qz + qx*qy),qw^2 + qx^2 - qy^2 - qz^2);
    if((currentAngle < -pi) || (pi < currentAngle))
        currentAngle = mod(currentAngle+pi, 2*pi)-pi;
    end
    vel_x = vx;
    vel_y = vy;
    
    q = quaternion(qw, qx, qy, qy);
    dt = 0.001;
    av = angvel(q, dt,'frame');
    w_meas = av(3);
    rotated_path = path; 
end

== matlab function SSMM_sim_Torque_3DOF/HBZ Controller/MATLAB Function4 ==
  data: u input; v output; waypoints input; rotation output; stop output
function [v, rotation, stop] = HBZ(u, waypoints)
%-------------------Persistent Variable Initialization--------------------%
persistent delta_old;
persistent path_ind;
persistent pathlength;
persistent pathPre;
persistent path;
persistent delta;
persistent old_theta;

if isempty(path_ind)
    delta_old = 0;
    delta = 0;
    path_ind = 1;
    pathPre=waypoints;
    [pathlength,~]=size(pathPre);  
   path=[pathPre; pathPre(pathlength,1)+100 pathPre(pathlength,2)+100]; %sim takes multiple iterations to stop after reaching final point, so this prevents it from breaking
end
    
%----------------------Vehicle/ Controller Parameters---------------------%
k1 = 8.0;
k2 = 40.0;
lambda = 2.0;
theta_a = pi/8;
x_ICR = 0.0;
y_ICR_l = 0.2812;
y_ICR_r = -0.2812;
alpha_l = 1.022;
alpha_r = 1.022;
epsilon = 0.5;
max_angular_velocity = 4.0;
Vm = 2.0;
Ts = 0.001;

%---------------------Geometry Related To The Vehicle---------------------%
x_meas = u(1);
y_meas = u(2);
theta_meas = u(3);

R = [cos(theta_meas), -sin(theta_meas);
     sin(theta_meas),  cos(theta_meas)];

v_local = R * [u(4); u(5)];
v_local_x_meas = v_local(1) * sign(v_local(1));

if isempty(old_theta)
    angular_vel_meas = 0;
    old_theta = 0;
else
    angular_vel_meas = (theta_meas - old_theta)/Ts;
    old_theta = u(3);
end


Vl = (v_local_x_meas - y_ICR_l * angular_vel_meas)/alpha_l;
Vr = (v_local_x_meas - y_ICR_r * angular_vel_meas)/alpha_r;
Vl = clamp(Vl, 0, Vm);
Vr = clamp(Vr, 0, Vm);

if(Vl == 0 & Vr == 0)
    curvature = 0;
else
    curvature = (alpha_r * Vr - alpha_l * Vl)/...
        sqrt(( alpha_r*y_ICR_l*Vr - alpha_l*y_ICR_r*Vl)^2 + ...
             (-alpha_r*x_ICR  *Vr + alpha_l*x_ICR  *Vl)^2)
end     
%--------------------Geometry Related To The Waypoint---------------------%
pos=[u(1) u(2)]; % [x,y] 
currentPoint=path(path_ind,:);
target=path(path_ind+1,:);

Px = target(1);
Py = target(2);
theta_p = atan2(target(2)-currentPoint(2), (target(1)-currentPoint(1)));

theta_p = angleClamp(theta_p);

%----------------------Vehicle Errors To The Waypoint---------------------%   
% Robot position vector module
r = hypot(x_meas - Px, y_meas - Py);

% Robot position vector angle in world coordinates
theta_r = atan2(y_meas - Py, x_meas - Px);

% Robot position vector angle in path coordinates
delta_theta = AngleDelta(theta_p, theta_r);

% Current robot position in path coordinates
xe = r * cos(delta_theta);
ye = r * sin(delta_theta);

% Calculate theta_e
theta_e = AngleDelta(theta_p,theta_meas);

%------------------------------Speed Command------------------------------% 
v = Vm;

V1 = 1/2 * (xe^2 + ye^2 + 1/lambda * abs(sin(theta_e - delta)));

if angular_vel_meas > 0
    if V1 >= epsilon
        v = (-alpha_r * y_ICR_l * Vm) / (y_ICR_r - y_ICR_l)
    elseif V1 < epsilon
        v = (alpha_r * Vm) / (1 + abs(y_ICR_r * curvature))
    end
elseif angular_vel_meas <= 0
    if V1 >= epsilon
        v = (alpha_l * y_ICR_r * Vm) / (y_ICR_r - y_ICR_l)
    elseif V1 < epsilon
        v = (alpha_l * Vm) / (1 + abs(y_ICR_l * curvature))
    end
end

%-----------------------------Steering Command----------------------------% 
delta_old = delta;
delta = AngleClamp(-theta_a * tanh(ye));
delta_prim = (delta - delta_old) / Ts;

%%%%%% MIGHT NEED TO ADD EXPONENTIAL SPEED CONTROL FACTOR %%%%%
%exp_factor = computeSpeedControl();
%v = v * exp_factor;

theta_diff = AngleDelta(delta, theta_e);

trig_ratio = (abs(sin(theta_diff))) / (sin(theta_diff) * cos(theta_diff));
theta_e_prim = delta_prim ...
        - lambda * trig_ratio * ye * v * sin(theta_e) ...
        + lambda * trig_ratio * ye * x_ICR * angular_vel_meas * cos(theta_e) ...
        - k2 * trig_ratio * theta_diff * theta_diff;

% Calculate the speed of the "virtual vehicle"
s_prim = v * cos(theta_e) + x_ICR * angular_vel_meas * sin(theta_e) + k1 * xe;

if s_prim < 0
    s_prim = 0; 
end

omega = theta_e_prim + curvature * s_prim;
rotation = clamp(omega, -max_angular_velocity, max_angular_velocity);

%-----------------------------Update Waypoint-----------------------------%
A = [(currentPoint(2)-target(2)), target(1)-currentPoint(1); target(1)-currentPoint(1), target(2)-currentPoint(2)];
b = [ target(1)*currentPoint(2)-currentPoint(1)*target(2); pos(1)*(target(1)-currentPoint(1)) + pos(2)*(target(2)-currentPoint(2))];
proj = (A\b)'; %projected point on the line between  .
projLen=dot(proj-currentPoint,target-currentPoint)/norm(target-currentPoint)^2; %the distance along the projected line, where 0 is the start point and 1 is the end point

if ((projLen>1))
    path_ind=path_ind+1;
end

%check if at destination and terminate sim if there
pathflag=0;
if (path_ind==pathlength)
    pathflag=1;
end
stop = pathflag;

%----------------------------Helper Functions-----------------------------%
function theta_out = angleClamp(theta_in)
    if((theta_in < -pi) || (pi < theta_in)) % wrap to +/-pi
        theta_out = mod(theta_in+pi, 2*pi)-pi;
    else
        theta_out = theta_in;
    end
end
function x = clamp(x, lower, upper)
    x = max(min(x, upper), lower);
end
function out      = AngleClamp(angleRad)
    M_PI = pi;  % MATLAB uses 'pi' for the value of π
    out = angleRad;
    
    while out < -M_PI
        out = out + 2 * M_PI;
    end

    while out >= M_PI
        out = out - 2 * M_PI;
    end
end
function [ret] = AngleDelta(a1, a2)
    M_PI = pi;  % MATLAB uses 'pi' for the value of π

    ret = a2 - a1;

    while ret > M_PI
        ret = ret - 2.0 * M_PI;
    end

    while ret < -M_PI
        ret = ret + 2.0 * M_PI;
    end
end
end

== matlab function SSMM_sim_Torque_3DOF/Pure Pursuit Controller/MATLAB Function ==
  data: u input; y output
function y = fcn(u)
%jackal dyanamic model

pos=[u(1) u(2)]; % [x,y]
currentAngle=u(3);
y = [pos currentAngle];

== matlab function SSMM_sim_Torque_3DOF/Fuzzy Controller/Fuzzy Errors ==
  settings: updateMethod=DISCRETE
  data: u input; y output
function y  = fcn(u)

kLOOK = 0.95;

pos = [u(1), u(2)];
currentAngle = u(3);
currentPoint=[u(4) u(5)];
target=[u(6) u(7)];
future=[u(8) u(9)];

A = [(currentPoint(2)-target(2)), target(1)-currentPoint(1); target(1)-currentPoint(1), target(2)-currentPoint(2)];
b = [ target(1)*currentPoint(2)-currentPoint(1)*target(2); pos(1)*(target(1)-currentPoint(1)) + pos(2)*(target(2)-currentPoint(2))];
proj = (A\b)'; %projected point on the line between  .

d = ( pos(1)-currentPoint(1) )*(target(2)-currentPoint(2)) - (pos(2)-currentPoint(2))*(target(1)-currentPoint(1));

if ( d >0)
    side = 1;
elseif ( d < 0)
    side = -1;
else
    side = 0;
end

distanceLine=norm(pos-proj)*side;
distanceTarget=sqrt((target(1)-pos(1))^2+(target(2)-pos(2))^2);

%wrap to +/-pi
if((currentAngle < -pi) || (pi < currentAngle))
    currentAngle = mod(currentAngle+pi, 2*pi)-pi;
end

farTarget=[kLOOK*proj(1)+(1-kLOOK)*target(1) kLOOK*proj(2)+(1-kLOOK)*target(2)];

th1 = atan2(farTarget(2)-pos(2), farTarget(1)-pos(1));
th2 = atan2(target(2)-currentPoint(2), target(1)-currentPoint(1));
th3 = atan2(future(2)-target(2), future(1)-target(1)); 

ThetaFar=th1-currentAngle;
ThetaNear=th2-currentAngle;
ThetaLookahead=th3-currentAngle;

%wrap to +/-pi
if((ThetaFar < -pi) || (pi < ThetaFar))
    ThetaFar = mod(ThetaFar+pi, 2*pi)-pi;
end

%wrap to +/-pi
if((ThetaNear < -pi) || (pi < ThetaNear))
    ThetaNear = mod(ThetaNear+pi, 2*pi)-pi;
end

%wrap to +/-pi
if((ThetaLookahead < -pi) || (pi < ThetaLookahead))
    ThetaLookahead = mod(ThetaLookahead+pi, 2*pi)-pi;
end

y = [distanceLine;ThetaFar;ThetaNear;ThetaLookahead;distanceTarget];

== matlab function SSMM_sim_Torque_3DOF/Fuzzy Controller/Target Signals Generator1 ==
  data: u1 input; y output; u2 input; stop output
function [y,stop] = fcn(u1,u2)
persistent pathcount;
persistent pathlength;
persistent path; %error in code, initially used path but this is already a matlab function
persistent pathPre;

if isempty(pathcount)
   pathcount=1;
   pathPre=u2;
   [pathlength,~]=size(pathPre);  
   path=[pathPre; pathPre(pathlength,1)+100 pathPre(pathlength,2)+100]; %sim takes multiple iterations to stop after reaching final point, so this prevents it from breaking
end

pos=[u1(1) u1(2)]; % [x,y] 
currentPoint=path(pathcount,:);
target=path(pathcount+1,:);

A = [(currentPoint(2)-target(2)), target(1)-currentPoint(1); target(1)-currentPoint(1), target(2)-currentPoint(2)];
b = [ target(1)*currentPoint(2)-currentPoint(1)*target(2); pos(1)*(target(1)-currentPoint(1)) + pos(2)*(target(2)-currentPoint(2))];
proj = (A\b)'; %projected point on the line between  .
projLen=dot(proj-currentPoint,target-currentPoint)/norm(target-currentPoint)^2; %the distance along the projected line, where 0 is the start point and 1 is the end point

if ((projLen>1))
    pathcount=pathcount+1;
end

%check if at destination and terminate sim if there
pathflag=0;
if (pathcount==pathlength)
    pathflag=1;
end

if ((pathcount==(pathlength-1))||(pathcount==(pathlength)))
    a=path(pathcount,:);
    b=path(pathcount+1,:);
    diff = (b-a) / norm(b-a);
    post = b + diff;
else
    a=path(pathcount,:);
    b=path(pathcount+1,:);
    post=path(pathcount+2,:);
end

y = [a(1);a(2);b(1);b(2);post(1);post(2)];
stop=pathflag;

== matlab function SSMM_sim_Torque_3DOF/Pure Pursuit Controller/Fuzzy Controller/Fuzzy Errors ==
  settings: updateMethod=DISCRETE
  data: u input; y output
function y  = fcn(u)
kLOOK = 0.95;

pos=[u(1) u(2)]; % [x,y]
currentAngle = u(3);
currentPoint=[u(4) u(5)];
target=[u(6) u(7)];
future=[u(8) u(9)];

A = [(currentPoint(2)-target(2)), target(1)-currentPoint(1); target(1)-currentPoint(1), target(2)-currentPoint(2)];
b = [ target(1)*currentPoint(2)-currentPoint(1)*target(2); pos(1)*(target(1)-currentPoint(1)) + pos(2)*(target(2)-currentPoint(2))];
proj = (A\b)'; %projected point on the line between  .

d = ( pos(1)-currentPoint(1) )*(target(2)-currentPoint(2)) - (pos(2)-currentPoint(2))*(target(1)-currentPoint(1));

if ( d >0)
    side = 1;
elseif ( d < 0)
    side = -1;
else
    side = 0;
end

distanceLine=norm(pos-proj)*side;
distanceTarget=sqrt((target(1)-pos(1))^2+(target(2)-pos(2))^2);

%wrap to +/-pi
if((currentAngle < -pi) || (pi < currentAngle))
    currentAngle = mod(currentAngle+pi, 2*pi)-pi;
end

farTarget=[kLOOK*proj(1)+(1-kLOOK)*target(1) kLOOK*proj(2)+(1-kLOOK)*target(2)];

th1 = atan2(farTarget(2)-pos(2), farTarget(1)-pos(1));
th2 = atan2(target(2)-currentPoint(2), target(1)-currentPoint(1));
th3 = atan2(future(2)-target(2), future(1)-target(1)); 

ThetaFar=th1-currentAngle;
ThetaNear=th2-currentAngle;
ThetaLookahead=th3-currentAngle;

%wrap to +/-pi
if((ThetaFar < -pi) || (pi < ThetaFar))
    ThetaFar = mod(ThetaFar+pi, 2*pi)-pi;
end

%wrap to +/-pi
if((ThetaNear < -pi) || (pi < ThetaNear))
    ThetaNear = mod(ThetaNear+pi, 2*pi)-pi;
end

%wrap to +/-pi
if((ThetaLookahead < -pi) || (pi < ThetaLookahead))
    ThetaLookahead = mod(ThetaLookahead+pi, 2*pi)-pi;
end

y = [distanceLine;ThetaFar;ThetaNear;ThetaLookahead;distanceTarget];

== matlab function SSMM_sim_Torque_3DOF/Pure Pursuit Controller/Fuzzy Controller/Target Signals Generator1 ==
  data: u1 input; y output; u2 input; stop output
function [y,stop] = fcn(u1,u2)
persistent pathcount;
persistent pathlength;
persistent path; %error in code, initially used path but this is already a matlab function
persistent pathPre;

if isempty(pathcount)
   pathcount=1;
   pathPre=u2;
   [pathlength,~]=size(pathPre);  
   path=[pathPre; pathPre(pathlength,1)+100 pathPre(pathlength,2)+100]; %sim takes multiple iterations to stop after reaching final point, so this prevents it from breaking
end


pos=[u1(1) u1(2)]; % [x,y] 
currentPoint=path(pathcount,:);
target=path(pathcount+1,:);

A = [(currentPoint(2)-target(2)), target(1)-currentPoint(1); target(1)-currentPoint(1), target(2)-currentPoint(2)];
b = [ target(1)*currentPoint(2)-currentPoint(1)*target(2); pos(1)*(target(1)-currentPoint(1)) + pos(2)*(target(2)-currentPoint(2))];
proj = (A\b)'; %projected point on the line between  .
projLen=dot(proj-currentPoint,target-currentPoint)/norm(target-currentPoint)^2; %the distance along the projected line, where 0 is the start point and 1 is the end point

if ((projLen>1))
    pathcount=pathcount+1;
end

%check if at destination and terminate sim if there
pathflag=0;
if (pathcount==pathlength)
    pathflag=1;
end

if ((pathcount==(pathlength-1))||(pathcount==(pathlength)))
    a=path(pathcount,:);
    b=path(pathcount+1,:);
    diff = (b-a) / norm(b-a);
    post = b + diff;
else
    a=path(pathcount,:);
    b=path(pathcount+1,:);
    post=path(pathcount+2,:);
end

y = [a(1);a(2);b(1);b(2);post(1);post(2)];
stop=pathflag;

== matlab function SSMM_sim_Torque_3DOF/Fuzzy Controller/MATLAB Function ==
  data: pos_x output; pos_y output; qw input; currentAngle output; qx input; qy input; qz input; px input; py input; path input; rotated_path output
function [pos_x, pos_y, currentAngle, rotated_path] = fcn(qw, qx, qy, qz, px, py, path)
    pos_x = px;
    pos_y = py;
    currentAngle = atan2(2*(qw*qz + qx*qy),1-2*(qy^2 + qz^2));
    if((currentAngle < -pi) || (pi < currentAngle))
        currentAngle = mod(currentAngle+pi, 2*pi)-pi;
    end
    rotated_path = path; 
end

== matlab function SSMM_sim_Torque_3DOF/Pure Pursuit Controller/MATLAB Function1 ==
  data: pos_x output; pos_y output; qw input; currentAngle output; qx input; qy input; qz input; px input; py input; path input; rotated_path output
function [pos_x, pos_y, currentAngle, rotated_path] = fcn(qw, qx, qy, qz, px, py, path)
    pos_x = px;
    pos_y = py;
    currentAngle = atan2(2*(qw*qz + qx*qy),1-2*(qy^2 + qz^2));
    if((currentAngle < -pi) || (pi < currentAngle))
        currentAngle = mod(currentAngle+pi, 2*pi)-pi;
    end
    rotated_path = path; 
end

== matlab function SSMM_sim_Torque_3DOF/HBZ Controller/Fuzzy Controller1/Fuzzy Errors ==
  settings: updateMethod=DISCRETE
  data: u input; y output
function y  = fcn(u)
kLOOK = 0.95;

pos=[u(1) u(2)]; % [x,y]
currentAngle = u(3);
currentPoint=[u(7) u(8)];
target=[u(9) u(10)];
future=[u(11) u(12)];

A = [(currentPoint(2)-target(2)), target(1)-currentPoint(1); target(1)-currentPoint(1), target(2)-currentPoint(2)];
b = [ target(1)*currentPoint(2)-currentPoint(1)*target(2); pos(1)*(target(1)-currentPoint(1)) + pos(2)*(target(2)-currentPoint(2))];
proj = (A\b)'; %projected point on the line between  .

d = ( pos(1)-currentPoint(1) )*(target(2)-currentPoint(2)) - (pos(2)-currentPoint(2))*(target(1)-currentPoint(1));

if ( d >0)
    side = 1;
elseif ( d < 0)
    side = -1;
else
    side = 0;
end

distanceLine=norm(pos-proj)*side;
distanceTarget=sqrt((target(1)-pos(1))^2+(target(2)-pos(2))^2);

%wrap to +/-pi
if((currentAngle < -pi) || (pi < currentAngle))
    currentAngle = mod(currentAngle+pi, 2*pi)-pi;
end

farTarget=[kLOOK*proj(1)+(1-kLOOK)*target(1) kLOOK*proj(2)+(1-kLOOK)*target(2)];

th1 = atan2(farTarget(2)-pos(2), farTarget(1)-pos(1));
th2 = atan2(target(2)-currentPoint(2), target(1)-currentPoint(1));
th3 = atan2(future(2)-target(2), future(1)-target(1)); 

ThetaFar=th1-currentAngle;
ThetaNear=th2-currentAngle;
ThetaLookahead=th3-currentAngle;

%wrap to +/-pi
if((ThetaFar < -pi) || (pi < ThetaFar))
    ThetaFar = mod(ThetaFar+pi, 2*pi)-pi;
end

%wrap to +/-pi
if((ThetaNear < -pi) || (pi < ThetaNear))
    ThetaNear = mod(ThetaNear+pi, 2*pi)-pi;
end

%wrap to +/-pi
if((ThetaLookahead < -pi) || (pi < ThetaLookahead))
    ThetaLookahead = mod(ThetaLookahead+pi, 2*pi)-pi;
end

y = [distanceLine;ThetaFar;ThetaNear;ThetaLookahead;distanceTarget];
